simulink model "model_reg_rik"  (R2024a)
settings: Solver=FixedStepAuto  StartTime=0.0  StopTime=10  FixedStep=0.0001  MinStep=1e-8  RelTol=1e-8  AbsTol=1e-8
model workspace (MAT data in the model file):
  A = [11  -2  13; 6  -1  6; -6  -1  -8]
  B = [2; 0; 0]
  K = [-4 2.4167 -3]
values from neighbouring files (symbols this model uses):
  K1_1 = Y*inv(P)    [reg1.m]
  K1_2 = Y*inv(P)    [reg2.m]
  K1_3 = Y*inv(P)    [reg3.m]
  K2_1 = Y*inv(P)    [reg_minimize1.m]
  K2_2 = Y*inv(P)    [reg_minimize2.m]
  K2_3 = Y*inv(P)    [reg_minimize3.m]
  K3_1 = -inv(R)*B'*P    [reg_rik1.m]
  K3_2 = -inv(R)*B'*P    [reg_rik2.m]
  K3_3 = -inv(R)*B'*P    [reg_rik3.m]
  K4_1 = -inv(R)*B'*P    [reg_rik_minimize1.m]
  K4_2 = -inv(R)*B'*P    [reg_rik_minimize2.m]
  K4_3 = -inv(R)*B'*P    [reg_rik_minimize3.m]
settings Model: Creator=ventus  LastModifiedBy=ventus

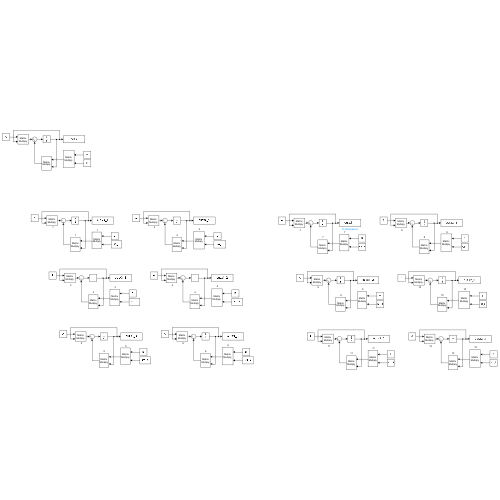
[thumbnail: Simulink's stored preview of the top-level diagram]
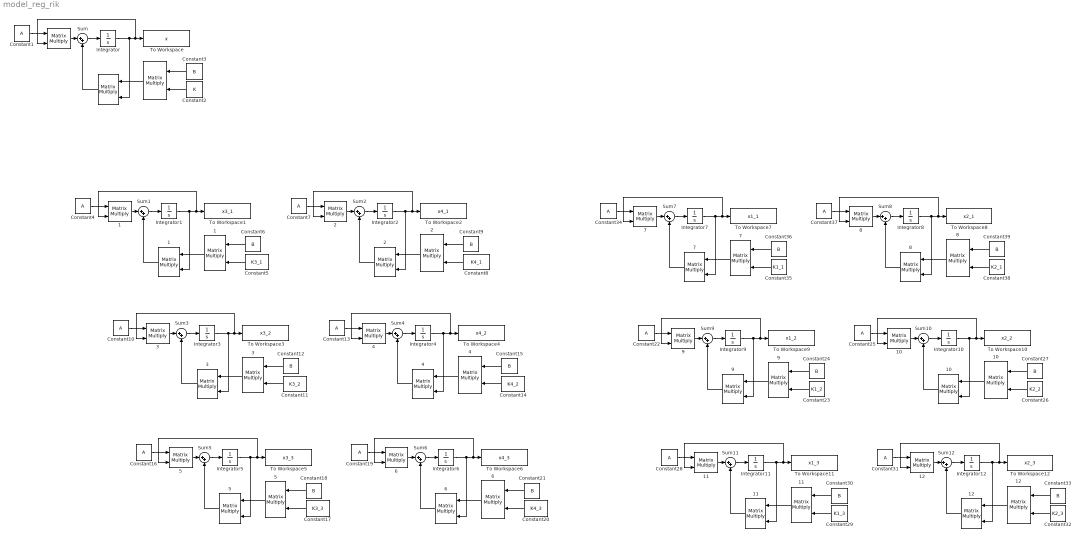
== system model_reg_rik ==
   {,1..12} (13 alike) : Product  Multiplication=Matrix(*)
    {,1..12} (13 alike) : Product  Multiplication=Matrix(*)
     {,1..12} (13 alike) : Product  Multiplication=Matrix(*)
  Constant{1,4,7,10,13,16,19,22,25,28,31,34,37} (13 alike) : Constant  Value=A  VectorParams1D=off
  Constant11 : Constant  Value=K3_2  VectorParams1D=off
  Constant{3,6,9,12,15,18,21,24,27,30,33,36,39} (13 alike) : Constant  Value=B  VectorParams1D=off
  Constant14 : Constant  Value=K4_2  VectorParams1D=off
  Constant17 : Constant  Value=K3_3  VectorParams1D=off
  Constant2 : Constant  Value=K  VectorParams1D=off
  Constant20 : Constant  Value=K4_3  VectorParams1D=off
  Constant23 : Constant  Value=K1_2  VectorParams1D=off
  Constant26 : Constant  Value=K2_2  VectorParams1D=off
  Constant29 : Constant  Value=K1_3  VectorParams1D=off
  Constant32 : Constant  Value=K2_3  VectorParams1D=off
  Constant35 : Constant  Value=K1_1  VectorParams1D=off
  Constant38 : Constant  Value=K2_1  VectorParams1D=off
  Constant5 : Constant  Value=K3_1  VectorParams1D=off
  Constant8 : Constant  Value=K4_1  VectorParams1D=off
  Integrator{,1..12} (13 alike) : Integrator  InitialCondition=[1; 1; 1]
  Sum{,1..12} (13 alike) : Sum  Inputs=|++
  To Workspace : ToWorkspace  VariableName=x  SaveFormat=Timeseries  SampleTime=-1
  To Workspace1 : ToWorkspace  VariableName=x3_1  SaveFormat=Timeseries  SampleTime=-1
  To Workspace10 : ToWorkspace  VariableName=x2_2  SaveFormat=Timeseries  SampleTime=-1
  To Workspace11 : ToWorkspace  VariableName=x1_3  SaveFormat=Timeseries  SampleTime=-1
  To Workspace12 : ToWorkspace  VariableName=x2_3  SaveFormat=Timeseries  SampleTime=-1
  To Workspace2 : ToWorkspace  VariableName=x4_1  SaveFormat=Timeseries  SampleTime=-1
  To Workspace3 : ToWorkspace  VariableName=x3_2  SaveFormat=Timeseries  SampleTime=-1
  To Workspace4 : ToWorkspace  VariableName=x4_2  SaveFormat=Timeseries  SampleTime=-1
  To Workspace5 : ToWorkspace  VariableName=x3_3  SaveFormat=Timeseries  SampleTime=-1
  To Workspace6 : ToWorkspace  VariableName=x4_3  SaveFormat=Timeseries  SampleTime=-1
  To Workspace7 : ToWorkspace  VariableName=x1_1  SaveFormat=Timeseries  SampleTime=-1
  To Workspace8 : ToWorkspace  VariableName=x2_1  SaveFormat=Timeseries  SampleTime=-1
  To Workspace9 : ToWorkspace  VariableName=x1_2  SaveFormat=Timeseries  SampleTime=-1
  wires:
  Integrator/1 -> To Workspace/1, "   "/2, " "/2
  Constant2/1 -> "  "/2
  "  "/1 -> " "/1
  " "/1 -> Sum/2
  Sum/1 -> Integrator/1
  Constant3/1 -> "  "/1
  Constant1/1 -> "   "/1
  "   "/1 -> Sum/1
  " 1"/1 -> Sum1/2
  Constant6/1 -> "  1"/1
  "  1"/1 -> " 1"/1
  "   1"/1 -> Sum1/1
  Sum1/1 -> Integrator1/1
  Constant4/1 -> "   1"/1
  Constant5/1 -> "  1"/2
  Integrator1/1 -> To Workspace1/1, "   1"/2, " 1"/2
  " 2"/1 -> Sum2/2
  Constant9/1 -> "  2"/1
  "  2"/1 -> " 2"/1
  "   2"/1 -> Sum2/1
  Sum2/1 -> Integrator2/1
  Constant7/1 -> "   2"/1
  Constant8/1 -> "  2"/2
  Integrator2/1 -> To Workspace2/1, "   2"/2, " 2"/2
  "  4"/1 -> " 4"/1
  Integrator3/1 -> To Workspace3/1, "   3"/2, " 3"/2
  Constant14/1 -> "  4"/2
  Integrator4/1 -> To Workspace4/1, "   4"/2, " 4"/2
  "   4"/1 -> Sum4/1
  "  3"/1 -> " 3"/1
  Constant13/1 -> "   4"/1
  " 3"/1 -> Sum3/2
  Constant15/1 -> "  4"/1
  "   3"/1 -> Sum3/1
  Sum4/1 -> Integrator4/1
  " 4"/1 -> Sum4/2
  Constant12/1 -> "  3"/1
  Constant11/1 -> "  3"/2
  Sum3/1 -> Integrator3/1
  Constant10/1 -> "   3"/1
  "  6"/1 -> " 6"/1
  Integrator5/1 -> To Workspace5/1, "   5"/2, " 5"/2
  Constant20/1 -> "  6"/2
  Integrator6/1 -> To Workspace6/1, "   6"/2, " 6"/2
  "   6"/1 -> Sum6/1
  "  5"/1 -> " 5"/1
  Constant19/1 -> "   6"/1
  " 5"/1 -> Sum5/2
  Constant21/1 -> "  6"/1
  "   5"/1 -> Sum5/1
  Sum6/1 -> Integrator6/1
  " 6"/1 -> Sum6/2
  Constant18/1 -> "  5"/1
  Constant17/1 -> "  5"/2
  Sum5/1 -> Integrator5/1
  Constant16/1 -> "   5"/1
  "  9"/1 -> " 9"/1
  Sum8/1 -> Integrator8/1
  " 8"/1 -> Sum8/2
  " 11"/1 -> Sum11/2
  Constant31/1 -> "   12"/1
  Constant26/1 -> "  10"/2
  Integrator9/1 -> To Workspace9/1, "   9"/2, " 9"/2
  Sum12/1 -> Integrator12/1
  "   11"/1 -> Sum11/1
  Constant33/1 -> "  12"/1
  Integrator11/1 -> To Workspace11/1, "   11"/2, " 11"/2
  Sum9/1 -> Integrator9/1
  "  11"/1 -> " 11"/1
  " 10"/1 -> Sum10/2
  Constant24/1 -> "  9"/1
  "   8"/1 -> Sum8/1
  Constant23/1 -> "  9"/2
  "  12"/1 -> " 12"/1
  Constant25/1 -> "   10"/1
  " 7"/1 -> Sum7/2
  " 9"/1 -> Sum9/2
  Constant34/1 -> "   7"/1
  "  10"/1 -> " 10"/1
  Constant32/1 -> "  12"/2
  Constant38/1 -> "  8"/2
  Constant37/1 -> "   8"/1
  "   10"/1 -> Sum10/1
  Integrator10/1 -> To Workspace10/1, "   10"/2, " 10"/2
  Integrator8/1 -> To Workspace8/1, "   8"/2, " 8"/2
  Constant39/1 -> "  8"/1
  "   9"/1 -> Sum9/1
  "   7"/1 -> Sum7/1
  "  7"/1 -> " 7"/1
  Sum7/1 -> Integrator7/1
  Integrator12/1 -> To Workspace12/1, "   12"/2, " 12"/2
  "  8"/1 -> " 8"/1
  Integrator7/1 -> To Workspace7/1, "   7"/2, " 7"/2
  " 12"/1 -> Sum12/2
  Constant29/1 -> "  11"/2
  Constant35/1 -> "  7"/2
  "   12"/1 -> Sum12/1
  Constant27/1 -> "  10"/1
  Constant30/1 -> "  11"/1
  Constant28/1 -> "   11"/1
  Constant22/1 -> "   9"/1
  Constant36/1 -> "  7"/1
  Sum11/1 -> Integrator11/1
  Sum10/1 -> Integrator10/1
